simulink model "test"  (Simulink 7.5)
settings: Solver=ode45  StartTime=0.0  StopTime=10.0  RelTol=1e-3
libraries: neural x103
settings Model: Creator=SAM-PC  LastModifiedBy=SAM-PC

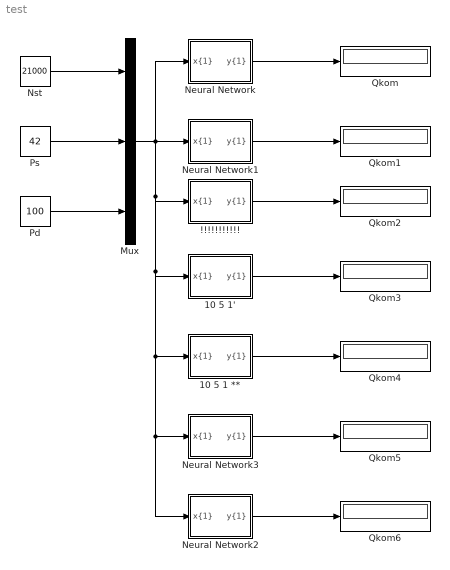
== system test ==
  !!!!!!!!!!! : Subsystem
  10 5 1 ** : Subsystem
  10 5 1' : Subsystem
  Mux : Mux  Inputs=3
  Neural Network : Subsystem
  Neural Network1 : Subsystem
  Neural Network2 : Subsystem
  Neural Network3 : Subsystem
  Nst : Constant  Value=21000  OutDataType=sfix(16)  OutScaling=2^0
  Pd : Constant  Value=100  OutDataType=sfix(16)  OutScaling=2^0
  Ps : Constant  Value=42  OutDataType=sfix(16)  OutScaling=2^0
  Qkom{,1..6} (7 alike) : Display
  wires:
  Mux/1 -> Neural Network/1("x{1}"), Neural Network1/1("x{1}"), !!!!!!!!!!!/1("x{1}"), 10 5 1'/1("x{1}"), 10 5 1 **/1("x{1}"), Neural Network3/1("x{1}"), Neural Network2/1("x{1}")
  Pd/1 -> Mux/3
  Ps/1 -> Mux/2
  Nst/1 -> Mux/1
  Neural Network/1("y{1}") -> Qkom/1
  Neural Network1/1("y{1}") -> Qkom1/1
  !!!!!!!!!!!/1("y{1}") -> Qkom2/1
  10 5 1'/1("y{1}") -> Qkom3/1
  10 5 1 **/1("y{1}") -> Qkom4/1
  Neural Network3/1("y{1}") -> Qkom5/1
  Neural Network2/1("y{1}") -> Qkom6/1

== system test/!!!!!!!!!!! ==
  "x{1}" : Inport  PortDimensions=3
  Layer 1 : Subsystem
  Layer 2 : Subsystem
  Process Input 1 : Subsystem
  Process Output 1 : Subsystem
  "y{1}" : Outport  InitialOutput=0
  wires:
  "x{1}"/1 -> Process Input 1/1(x)
  Process Output 1/1(y) -> "y{1}"/1
  Process Input 1/1(p) -> Layer 1/1("p{1}")
  Layer 1/1("a{1}") -> [feedback1]
  [feedback1] -> Layer 2/1("a{1} ")
  Layer 2/1("a{2}") -> Process Output 1/1(a)

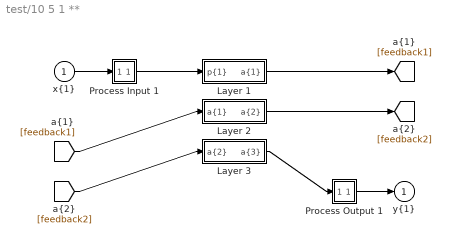
== system test/10 5 1 ** ==
  "x{1}" : Inport  PortDimensions=3
  Layer 1 : Subsystem
  Layer 2 : Subsystem
  Layer 3 : Subsystem
  Process Input 1 : Subsystem
  Process Output 1 : Subsystem
  "y{1}" : Outport  InitialOutput=0
  wires:
  Layer 3/1("a{3}") -> Process Output 1/1(a)
  [feedback2] -> Layer 3/1("a{2} ")
  Layer 2/1("a{2}") -> [feedback2]
  [feedback1] -> Layer 2/1("a{1} ")
  Layer 1/1("a{1}") -> [feedback1]
  Process Input 1/1(p) -> Layer 1/1("p{1}")
  Process Output 1/1(y) -> "y{1}"/1
  "x{1}"/1 -> Process Input 1/1(x)

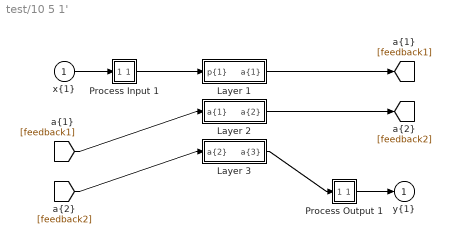
== system test/10 5 1' ==
  "x{1}" : Inport  PortDimensions=3
  Layer 1 : Subsystem
  Layer 2 : Subsystem
  Layer 3 : Subsystem
  Process Input 1 : Subsystem
  Process Output 1 : Subsystem
  "y{1}" : Outport  InitialOutput=0
  wires:
  Layer 3/1("a{3}") -> Process Output 1/1(a)
  [feedback2] -> Layer 3/1("a{2} ")
  Layer 2/1("a{2}") -> [feedback2]
  [feedback1] -> Layer 2/1("a{1} ")
  Layer 1/1("a{1}") -> [feedback1]
  Process Input 1/1(p) -> Layer 1/1("p{1}")
  Process Output 1/1(y) -> "y{1}"/1
  "x{1}"/1 -> Process Input 1/1(x)

== system test/Neural Network ==
  "x{1}" : Inport  PortDimensions=3
  Layer 1 : Subsystem
  Layer 2 : Subsystem
  Process Input 1 : Subsystem
  Process Output 1 : Subsystem
  "y{1}" : Outport  InitialOutput=0
  wires:
  "x{1}"/1 -> Process Input 1/1(x)
  Process Output 1/1(y) -> "y{1}"/1
  Process Input 1/1(p) -> Layer 1/1("p{1}")
  Layer 1/1("a{1}") -> [feedback1]
  [feedback1] -> Layer 2/1("a{1} ")
  Layer 2/1("a{2}") -> Process Output 1/1(a)

== system test/Neural Network1 ==
  "x{1}" : Inport  PortDimensions=3
  Layer 1 : Subsystem
  Layer 2 : Subsystem
  Process Input 1 : Subsystem
  Process Output 1 : Subsystem
  "y{1}" : Outport  InitialOutput=0
  wires:
  "x{1}"/1 -> Process Input 1/1(x)
  Process Output 1/1(y) -> "y{1}"/1
  Process Input 1/1(p) -> Layer 1/1("p{1}")
  Layer 1/1("a{1}") -> [feedback1]
  [feedback1] -> Layer 2/1("a{1} ")
  Layer 2/1("a{2}") -> Process Output 1/1(a)

== system test/Neural Network2 ==
  "x{1}" : Inport  PortDimensions=3
  Layer 1 : Subsystem
  Layer 2 : Subsystem
  Process Input 1 : Subsystem
  Process Output 1 : Subsystem
  "y{1}" : Outport  InitialOutput=0
  wires:
  Layer 2/1("a{2}") -> Process Output 1/1(a)
  [feedback1] -> Layer 2/1("a{1} ")
  Layer 1/1("a{1}") -> [feedback1]
  Process Input 1/1(p) -> Layer 1/1("p{1}")
  Process Output 1/1(y) -> "y{1}"/1
  "x{1}"/1 -> Process Input 1/1(x)

== system test/Neural Network3 ==
  "x{1}" : Inport  PortDimensions=3
  Layer 1 : Subsystem
  Layer 2 : Subsystem
  Process Input 1 : Subsystem
  Process Output 1 : Subsystem
  "y{1}" : Outport  InitialOutput=0
  wires:
  Layer 2/1("a{2}") -> Process Output 1/1(a)
  [feedback1] -> Layer 2/1("a{1} ")
  Layer 1/1("a{1}") -> [feedback1]
  Process Input 1/1(p) -> Layer 1/1("p{1}")
  Process Output 1/1(y) -> "y{1}"/1
  "x{1}"/1 -> Process Input 1/1(x)

== system test/!!!!!!!!!!!/Layer 1 ==
  "p{1}" : Inport  PortDimensions=3
  Delays 1 : Subsystem
      mask Display: disp('TDL')
  "IW{1,1}" : Subsystem
      mask Display: disp('weight')
  "b{1}" : Constant  Value=[-6.6059587578557615;-4.3526093218402542;-9.6125377715099489;15.34654034935151;-10.41504843932894;15.297045460594161;-11.215883022458025;-4.7902903485636283;-4.7770801252432253;-1.8726623455616338]
      mask Display: disp('bias')
  netsum : Sum  Inputs=2  OutDataType=sfix(16)  OutScaling=2^0  SaturateOnIntegerOverflow=on  InputSameDT=on  OutDataTypeStr=Inherit: Same as first input
  tansig : neural/Transfer Functions/tansig  SystemSampleTime=-1
  "a{1}" : Outport  InitialOutput=[0;0;0;0;0;0;0;0;0;0]
  wires:
  "p{1}"/1 -> Delays 1/1("p{1}")
  Delays 1/1("pd{1,1}") -> "IW{1,1}"/1("pd{1,1}")
  "IW{1,1}"/1("iz{1,1}") -> netsum/1
  "b{1}"/1 -> netsum/2
  netsum/1 -> tansig/1
  tansig/1 -> "a{1}"/1

== system test/!!!!!!!!!!!/Layer 2 ==
  "a{1} " : Inport  PortDimensions=10
  Delays 1 : Subsystem
      mask Display: disp('TDL')
  "LW{2,1}" : Subsystem
      mask Display: disp('weight')
  "b{2}" : Constant  Value=0.25321147312764225
      mask Display: disp('bias')
  netsum : Sum  Inputs=2  OutDataType=sfix(16)  OutScaling=2^0  SaturateOnIntegerOverflow=on  InputSameDT=on  OutDataTypeStr=Inherit: Same as first input
  purelin : neural/Transfer Functions/purelin  SystemSampleTime=-1
  "a{2}" : Outport  InitialOutput=0
  wires:
  "a{1} "/1 -> Delays 1/1("p{2}")
  Delays 1/1("pd{2,1}") -> "LW{2,1}"/1("ad{2,1}")
  "LW{2,1}"/1("lz{2,1}") -> netsum/1
  "b{2}"/1 -> netsum/2
  netsum/1 -> purelin/1
  purelin/1 -> "a{2}"/1

== system test/!!!!!!!!!!!/Process Input 1 ==
  x : Inport  PortDimensions=3
  p : Outport  PortDimensions=3
  wires:
  x/1 -> p/1

== system test/!!!!!!!!!!!/Process Output 1 ==
  a : Inport  PortDimensions=1
  y : Outport  PortDimensions=1
  wires:
  a/1 -> y/1

== system test/10 5 1 **/Layer 1 ==
  "p{1}" : Inport  PortDimensions=3
  Delays 1 : Subsystem
      mask Display: disp('TDL')
  "IW{1,1}" : Subsystem
      mask Display: disp('weight')
  "b{1}" : Constant  Value=[15.02277102392976;-1.3070946494642188;25.056968170821065;1.5453975487445806;-0.48029688944254451;5.9693538654521783;7.7677013128534886;-4.9232036490574114;-12.41463739376492;0.1231144148821651]
      mask Display: disp('bias')
  netsum : Sum  Inputs=2  OutDataType=sfix(16)  OutScaling=2^0  SaturateOnIntegerOverflow=on  InputSameDT=on  OutDataTypeStr=Inherit: Same as first input
  tansig : neural/Transfer Functions/tansig  SystemSampleTime=-1
  "a{1}" : Outport  InitialOutput=[0;0;0;0;0;0;0;0;0;0]
  wires:
  tansig/1 -> "a{1}"/1
  netsum/1 -> tansig/1
  "b{1}"/1 -> netsum/2
  "IW{1,1}"/1("iz{1,1}") -> netsum/1
  Delays 1/1("pd{1,1}") -> "IW{1,1}"/1("pd{1,1}")
  "p{1}"/1 -> Delays 1/1("p{1}")

== system test/10 5 1 **/Layer 2 ==
  "a{1} " : Inport  PortDimensions=10
  Delays 1 : Subsystem
      mask Display: disp('TDL')
  "LW{2,1}" : Subsystem
      mask Display: disp('weight')
  "b{2}" : Constant  Value=[2.8247030289932828;-7.9344890622783693;-8.5564708148276107;2.9733715127865676;6.28273195654105]
      mask Display: disp('bias')
  netsum : Sum  Inputs=2  OutDataType=sfix(16)  OutScaling=2^0  SaturateOnIntegerOverflow=on  InputSameDT=on  OutDataTypeStr=Inherit: Same as first input
  tansig : neural/Transfer Functions/tansig  SystemSampleTime=-1
  "a{2}" : Outport  InitialOutput=[0;0;0;0;0]
  wires:
  tansig/1 -> "a{2}"/1
  netsum/1 -> tansig/1
  "b{2}"/1 -> netsum/2
  "LW{2,1}"/1("lz{2,1}") -> netsum/1
  Delays 1/1("pd{2,1}") -> "LW{2,1}"/1("ad{2,1}")
  "a{1} "/1 -> Delays 1/1("p{2}")

== system test/10 5 1 **/Layer 3 ==
  "a{2} " : Inport  PortDimensions=5
  Delays 1 : Subsystem
      mask Display: disp('TDL')
  "LW{3,2}" : Subsystem
      mask Display: disp('weight')
  "b{3}" : Constant  Value=0.30034208922808647
      mask Display: disp('bias')
  netsum : Sum  Inputs=2  OutDataType=sfix(16)  OutScaling=2^0  SaturateOnIntegerOverflow=on  InputSameDT=on  OutDataTypeStr=Inherit: Same as first input
  purelin : neural/Transfer Functions/purelin  SystemSampleTime=-1
  "a{3}" : Outport  InitialOutput=0
  wires:
  purelin/1 -> "a{3}"/1
  netsum/1 -> purelin/1
  "b{3}"/1 -> netsum/2
  "LW{3,2}"/1("lz{3,2}") -> netsum/1
  Delays 1/1("pd{3,2}") -> "LW{3,2}"/1("ad{3,2}")
  "a{2} "/1 -> Delays 1/1("p{3}")

== system test/10 5 1 **/Process Input 1 ==
  x : Inport  PortDimensions=3
  p : Outport  PortDimensions=3
  wires:
  x/1 -> p/1

== system test/10 5 1 **/Process Output 1 ==
  a : Inport  PortDimensions=1
  y : Outport  PortDimensions=1
  wires:
  a/1 -> y/1

== system test/10 5 1'/Layer 1 ==
  "p{1}" : Inport  PortDimensions=3
  Delays 1 : Subsystem
      mask Display: disp('TDL')
  "IW{1,1}" : Subsystem
      mask Display: disp('weight')
  "b{1}" : Constant  Value=[18.413579066262386;13.657316243075135;18.043767679185159;11.250334678262735;3.5241900842698204;13.404243407569995;2.2257807010437509;9.6566319022558904;-3.0274634325673926;-4.0023507151100919]
      mask Display: disp('bias')
  netsum : Sum  Inputs=2  OutDataType=sfix(16)  OutScaling=2^0  SaturateOnIntegerOverflow=on  InputSameDT=on  OutDataTypeStr=Inherit: Same as first input
  tansig : neural/Transfer Functions/tansig  SystemSampleTime=-1
  "a{1}" : Outport  InitialOutput=[0;0;0;0;0;0;0;0;0;0]
  wires:
  tansig/1 -> "a{1}"/1
  netsum/1 -> tansig/1
  "b{1}"/1 -> netsum/2
  "IW{1,1}"/1("iz{1,1}") -> netsum/1
  Delays 1/1("pd{1,1}") -> "IW{1,1}"/1("pd{1,1}")
  "p{1}"/1 -> Delays 1/1("p{1}")

== system test/10 5 1'/Layer 2 ==
  "a{1} " : Inport  PortDimensions=10
  Delays 1 : Subsystem
      mask Display: disp('TDL')
  "LW{2,1}" : Subsystem
      mask Display: disp('weight')
  "b{2}" : Constant  Value=[2.1532494058916414;-0.67401500656272084;0.59110621272557129;-0.67490370527186982;1.3792550590079387]
      mask Display: disp('bias')
  netsum : Sum  Inputs=2  OutDataType=sfix(16)  OutScaling=2^0  SaturateOnIntegerOverflow=on  InputSameDT=on  OutDataTypeStr=Inherit: Same as first input
  tansig : neural/Transfer Functions/tansig  SystemSampleTime=-1
  "a{2}" : Outport  InitialOutput=[0;0;0;0;0]
  wires:
  tansig/1 -> "a{2}"/1
  netsum/1 -> tansig/1
  "b{2}"/1 -> netsum/2
  "LW{2,1}"/1("lz{2,1}") -> netsum/1
  Delays 1/1("pd{2,1}") -> "LW{2,1}"/1("ad{2,1}")
  "a{1} "/1 -> Delays 1/1("p{2}")

== system test/10 5 1'/Layer 3 ==
  "a{2} " : Inport  PortDimensions=5
  Delays 1 : Subsystem
      mask Display: disp('TDL')
  "LW{3,2}" : Subsystem
      mask Display: disp('weight')
  "b{3}" : Constant  Value=1.1366411649250561
      mask Display: disp('bias')
  netsum : Sum  Inputs=2  OutDataType=sfix(16)  OutScaling=2^0  SaturateOnIntegerOverflow=on  InputSameDT=on  OutDataTypeStr=Inherit: Same as first input
  purelin : neural/Transfer Functions/purelin  SystemSampleTime=-1
  "a{3}" : Outport  InitialOutput=0
  wires:
  purelin/1 -> "a{3}"/1
  netsum/1 -> purelin/1
  "b{3}"/1 -> netsum/2
  "LW{3,2}"/1("lz{3,2}") -> netsum/1
  Delays 1/1("pd{3,2}") -> "LW{3,2}"/1("ad{3,2}")
  "a{2} "/1 -> Delays 1/1("p{3}")

== system test/10 5 1'/Process Input 1 ==
  x : Inport  PortDimensions=3
  p : Outport  PortDimensions=3
  wires:
  x/1 -> p/1

== system test/10 5 1'/Process Output 1 ==
  a : Inport  PortDimensions=1
  y : Outport  PortDimensions=1
  wires:
  a/1 -> y/1

== system test/Neural Network/Layer 1 ==
  "p{1}" : Inport  PortDimensions=3
  Delays 1 : Subsystem
      mask Display: disp('TDL')
  "IW{1,1}" : Subsystem
      mask Display: disp('weight')
  "b{1}" : Constant  Value=[2.4324708557605383;-7.6739421539174089;3.0539465468465736;18.55085646224725;-23.635141756656115;-2.6793611692857526;17.680290988578996;-14.569548932519789;-13.842527653317914;-3.4475580624121687]
      mask Display: disp('bias')
  netsum : Sum  Inputs=2  OutDataType=sfix(16)  OutScaling=2^0  SaturateOnIntegerOverflow=on  InputSameDT=on  OutDataTypeStr=Inherit: Same as first input
  tansig : neural/Transfer Functions/tansig  SystemSampleTime=-1
  "a{1}" : Outport  InitialOutput=[0;0;0;0;0;0;0;0;0;0]
  wires:
  "p{1}"/1 -> Delays 1/1("p{1}")
  Delays 1/1("pd{1,1}") -> "IW{1,1}"/1("pd{1,1}")
  "IW{1,1}"/1("iz{1,1}") -> netsum/1
  "b{1}"/1 -> netsum/2
  netsum/1 -> tansig/1
  tansig/1 -> "a{1}"/1

== system test/Neural Network/Layer 2 ==
  "a{1} " : Inport  PortDimensions=10
  Delays 1 : Subsystem
      mask Display: disp('TDL')
  "LW{2,1}" : Subsystem
      mask Display: disp('weight')
  "b{2}" : Constant  Value=0.15810922780423164
      mask Display: disp('bias')
  netsum : Sum  Inputs=2  OutDataType=sfix(16)  OutScaling=2^0  SaturateOnIntegerOverflow=on  InputSameDT=on  OutDataTypeStr=Inherit: Same as first input
  purelin : neural/Transfer Functions/purelin  SystemSampleTime=-1
  "a{2}" : Outport  InitialOutput=0
  wires:
  "a{1} "/1 -> Delays 1/1("p{2}")
  Delays 1/1("pd{2,1}") -> "LW{2,1}"/1("ad{2,1}")
  "LW{2,1}"/1("lz{2,1}") -> netsum/1
  "b{2}"/1 -> netsum/2
  netsum/1 -> purelin/1
  purelin/1 -> "a{2}"/1

== system test/Neural Network/Process Input 1 ==
  x : Inport  PortDimensions=3
  p : Outport  PortDimensions=3
  wires:
  x/1 -> p/1

== system test/Neural Network/Process Output 1 ==
  a : Inport  PortDimensions=1
  y : Outport  PortDimensions=1
  wires:
  a/1 -> y/1

== system test/Neural Network1/Layer 1 ==
  "p{1}" : Inport  PortDimensions=3
  Delays 1 : Subsystem
      mask Display: disp('TDL')
  "IW{1,1}" : Subsystem
      mask Display: disp('weight')
  "b{1}" : Constant  Value=[-6.0166931774834991;-46.688706694529984;5.2999690825438703;18.493444026928799;-18.348040178794896;2.6103626315712543;-18.12090596934063;-7.1161048627161625;6.9740359095450248;-8.6996750974869972]
      mask Display: disp('bias')
  netsum : Sum  Inputs=2  OutDataType=sfix(16)  OutScaling=2^0  SaturateOnIntegerOverflow=on  InputSameDT=on  OutDataTypeStr=Inherit: Same as first input
  tansig : neural/Transfer Functions/tansig  SystemSampleTime=-1
  "a{1}" : Outport  InitialOutput=[0;0;0;0;0;0;0;0;0;0]
  wires:
  "p{1}"/1 -> Delays 1/1("p{1}")
  Delays 1/1("pd{1,1}") -> "IW{1,1}"/1("pd{1,1}")
  "IW{1,1}"/1("iz{1,1}") -> netsum/1
  "b{1}"/1 -> netsum/2
  netsum/1 -> tansig/1
  tansig/1 -> "a{1}"/1

== system test/Neural Network1/Layer 2 ==
  "a{1} " : Inport  PortDimensions=10
  Delays 1 : Subsystem
      mask Display: disp('TDL')
  "LW{2,1}" : Subsystem
      mask Display: disp('weight')
  "b{2}" : Constant  Value=-0.029512269905579976
      mask Display: disp('bias')
  netsum : Sum  Inputs=2  OutDataType=sfix(16)  OutScaling=2^0  SaturateOnIntegerOverflow=on  InputSameDT=on  OutDataTypeStr=Inherit: Same as first input
  purelin : neural/Transfer Functions/purelin  SystemSampleTime=-1
  "a{2}" : Outport  InitialOutput=0
  wires:
  "a{1} "/1 -> Delays 1/1("p{2}")
  Delays 1/1("pd{2,1}") -> "LW{2,1}"/1("ad{2,1}")
  "LW{2,1}"/1("lz{2,1}") -> netsum/1
  "b{2}"/1 -> netsum/2
  netsum/1 -> purelin/1
  purelin/1 -> "a{2}"/1

== system test/Neural Network1/Process Input 1 ==
  x : Inport  PortDimensions=3
  p : Outport  PortDimensions=3
  wires:
  x/1 -> p/1

== system test/Neural Network1/Process Output 1 ==
  a : Inport  PortDimensions=1
  y : Outport  PortDimensions=1
  wires:
  a/1 -> y/1

== system test/Neural Network2/Layer 1 ==
  "p{1}" : Inport  PortDimensions=3
  Delays 1 : Subsystem
      mask Display: disp('TDL')
  "IW{1,1}" : Subsystem
      mask Display: disp('weight')
  "b{1}" : Constant  Value=[15.912206318753258;7.7505120175037128;3.9018047854873212;-15.426996139049765;2.823989991488741;-11.93381184712964;-15.394961107894558;1.9154713229925484;-8.9241881256300211;-7.3222794371491178]
      mask Display: disp('bias')
  netsum : Sum  Inputs=2  OutDataType=sfix(16)  OutScaling=2^0  SaturateOnIntegerOverflow=on  InputSameDT=on  OutDataTypeStr=Inherit: Same as first input
  tansig : neural/Transfer Functions/tansig  SystemSampleTime=-1
  "a{1}" : Outport  InitialOutput=[0;0;0;0;0;0;0;0;0;0]
  wires:
  tansig/1 -> "a{1}"/1
  netsum/1 -> tansig/1
  "b{1}"/1 -> netsum/2
  "IW{1,1}"/1("iz{1,1}") -> netsum/1
  Delays 1/1("pd{1,1}") -> "IW{1,1}"/1("pd{1,1}")
  "p{1}"/1 -> Delays 1/1("p{1}")

== system test/Neural Network2/Layer 2 ==
  "a{1} " : Inport  PortDimensions=10
  Delays 1 : Subsystem
      mask Display: disp('TDL')
  "LW{2,1}" : Subsystem
      mask Display: disp('weight')
  "b{2}" : Constant  Value=0.97737461588991392
      mask Display: disp('bias')
  netsum : Sum  Inputs=2  OutDataType=sfix(16)  OutScaling=2^0  SaturateOnIntegerOverflow=on  InputSameDT=on  OutDataTypeStr=Inherit: Same as first input
  purelin : neural/Transfer Functions/purelin  SystemSampleTime=-1
  "a{2}" : Outport  InitialOutput=0
  wires:
  purelin/1 -> "a{2}"/1
  netsum/1 -> purelin/1
  "b{2}"/1 -> netsum/2
  "LW{2,1}"/1("lz{2,1}") -> netsum/1
  Delays 1/1("pd{2,1}") -> "LW{2,1}"/1("ad{2,1}")
  "a{1} "/1 -> Delays 1/1("p{2}")

== system test/Neural Network2/Process Input 1 ==
  x : Inport  PortDimensions=3
  p : Outport  PortDimensions=3
  wires:
  x/1 -> p/1

== system test/Neural Network2/Process Output 1 ==
  a : Inport  PortDimensions=1
  y : Outport  PortDimensions=1
  wires:
  a/1 -> y/1

== system test/Neural Network3/Layer 1 ==
  "p{1}" : Inport  PortDimensions=3
  Delays 1 : Subsystem
      mask Display: disp('TDL')
  "IW{1,1}" : Subsystem
      mask Display: disp('weight')
  "b{1}" : Constant  Value=[-22.415234115254385;-11.362832743815702;13.196213345352477;-23.274128799542019;-1.9079448236650758;5.6206820240612299;-14.499132702291242;-18.316509525440882;-16.167922059318332;-12.536388092109599]
      mask Display: disp('bias')
  netsum : Sum  Inputs=2  OutDataType=sfix(16)  OutScaling=2^0  SaturateOnIntegerOverflow=on  InputSameDT=on  OutDataTypeStr=Inherit: Same as first input
  tansig : neural/Transfer Functions/tansig  SystemSampleTime=-1
  "a{1}" : Outport  InitialOutput=[0;0;0;0;0;0;0;0;0;0]
  wires:
  tansig/1 -> "a{1}"/1
  netsum/1 -> tansig/1
  "b{1}"/1 -> netsum/2
  "IW{1,1}"/1("iz{1,1}") -> netsum/1
  Delays 1/1("pd{1,1}") -> "IW{1,1}"/1("pd{1,1}")
  "p{1}"/1 -> Delays 1/1("p{1}")

== system test/Neural Network3/Layer 2 ==
  "a{1} " : Inport  PortDimensions=10
  Delays 1 : Subsystem
      mask Display: disp('TDL')
  "LW{2,1}" : Subsystem
      mask Display: disp('weight')
  "b{2}" : Constant  Value=1.0819192782537284
      mask Display: disp('bias')
  netsum : Sum  Inputs=2  OutDataType=sfix(16)  OutScaling=2^0  SaturateOnIntegerOverflow=on  InputSameDT=on  OutDataTypeStr=Inherit: Same as first input
  purelin : neural/Transfer Functions/purelin  SystemSampleTime=-1
  "a{2}" : Outport  InitialOutput=0
  wires:
  purelin/1 -> "a{2}"/1
  netsum/1 -> purelin/1
  "b{2}"/1 -> netsum/2
  "LW{2,1}"/1("lz{2,1}") -> netsum/1
  Delays 1/1("pd{2,1}") -> "LW{2,1}"/1("ad{2,1}")
  "a{1} "/1 -> Delays 1/1("p{2}")

== system test/Neural Network3/Process Input 1 ==
  x : Inport  PortDimensions=3
  p : Outport  PortDimensions=3
  wires:
  x/1 -> p/1

== system test/Neural Network3/Process Output 1 ==
  a : Inport  PortDimensions=1
  y : Outport  PortDimensions=1
  wires:
  a/1 -> y/1

== system test/!!!!!!!!!!!/Layer 1/Delays 1 ==
  "p{1}" : Inport  PortDimensions=3
  mux : Mux  Inputs=1
  "pd{1,1}" : Outport
  wires:
  "p{1}"/1 -> mux/1
  mux/1 -> "pd{1,1}"/1

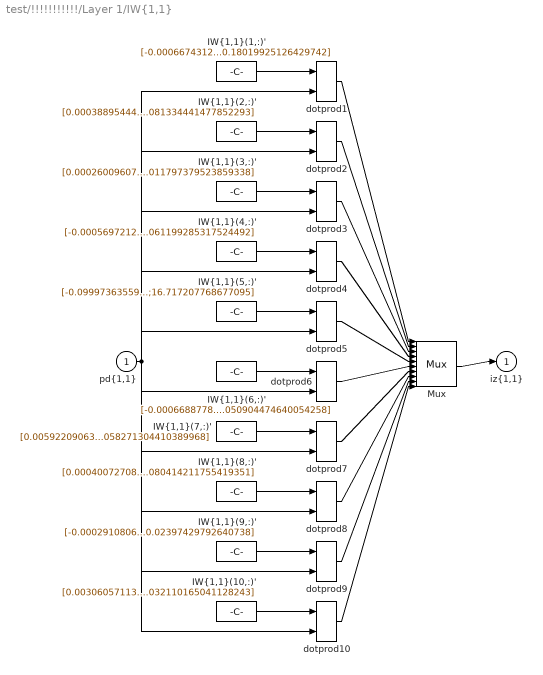
== system test/!!!!!!!!!!!/Layer 1/IW{1,1} ==
  "pd{1,1}" : Inport  PortDimensions=3
  "IW{1,1}(1,:)'" : Constant  Value=[-0.00066743122035897099;-0.11206446014488511;0.18019925126429742]
      mask Display: disp('weights')
  "IW{1,1}(10,:)'" : Constant  Value=[0.0030605711313751579;-0.096052630538237732;-0.032110165041128243]
      mask Display: disp('weights')
  "IW{1,1}(2,:)'" : Constant  Value=[0.0003889544485913661;0.15069729232506487;-0.081334441477852293]
      mask Display: disp('weights')
  "IW{1,1}(3,:)'" : Constant  Value=[0.00026009607440958632;0.063526490616979098;0.011797379523859338]
      mask Display: disp('weights')
  "IW{1,1}(4,:)'" : Constant  Value=[-0.00056972120462246755;-0.19132461828198041;0.061199285317524492]
      mask Display: disp('weights')
  "IW{1,1}(5,:)'" : Constant  Value=[-0.099973635598832711;2.8634131297756991;16.717207768677095]
      mask Display: disp('weights')
  "IW{1,1}(6,:)'" : Constant  Value=[-0.00066887787432494861;-0.18010598749241391;0.050904474640054258]
      mask Display: disp('weights')
  "IW{1,1}(7,:)'" : Constant  Value=[0.0059220906350217883;0.11468973909442041;-0.0058271304410389968]
      mask Display: disp('weights')
  "IW{1,1}(8,:)'" : Constant  Value=[0.00040072708699105176;0.15224871553489033;-0.080414211755419351]
      mask Display: disp('weights')
  "IW{1,1}(9,:)'" : Constant  Value=[-0.00029108067581634574;0.221865316933716;0.02397429792640738]
      mask Display: disp('weights')
  Mux : Mux  Inputs=10
  dotprod{1..10} (10 alike) : neural/Weight Functions/dotprod  SystemSampleTime=-1
  "iz{1,1}" : Outport
  wires:
  "IW{1,1}(1,:)'"/1 -> dotprod1/1
  "pd{1,1}"/1 -> dotprod1/2, dotprod2/2, dotprod3/2, dotprod4/2, dotprod5/2, dotprod6/2, dotprod7/2, dotprod8/2, dotprod9/2, dotprod10/2
  dotprod1/1 -> Mux/1
  "IW{1,1}(2,:)'"/1 -> dotprod2/1
  dotprod2/1 -> Mux/2
  "IW{1,1}(3,:)'"/1 -> dotprod3/1
  dotprod3/1 -> Mux/3
  "IW{1,1}(4,:)'"/1 -> dotprod4/1
  dotprod4/1 -> Mux/4
  "IW{1,1}(5,:)'"/1 -> dotprod5/1
  dotprod5/1 -> Mux/5
  "IW{1,1}(6,:)'"/1 -> dotprod6/1
  dotprod6/1 -> Mux/6
  "IW{1,1}(7,:)'"/1 -> dotprod7/1
  dotprod7/1 -> Mux/7
  "IW{1,1}(8,:)'"/1 -> dotprod8/1
  dotprod8/1 -> Mux/8
  "IW{1,1}(9,:)'"/1 -> dotprod9/1
  dotprod9/1 -> Mux/9
  "IW{1,1}(10,:)'"/1 -> dotprod10/1
  dotprod10/1 -> Mux/10
  Mux/1 -> "iz{1,1}"/1

== system test/!!!!!!!!!!!/Layer 2/Delays 1 ==
  "p{2}" : Inport  PortDimensions=10
  mux : Mux  Inputs=1
  "pd{2,1}" : Outport
  wires:
  "p{2}"/1 -> mux/1
  mux/1 -> "pd{2,1}"/1

== system test/!!!!!!!!!!!/Layer 2/LW{2,1} ==
  "ad{2,1}" : Inport  PortDimensions=10
  "IW{2,1}(1,:)'" : Constant  Value=[0.2014952594481072;-17.665856907001295;0.32895145996666803;-0.16313906729449315;-0.010968372198123189;-0.16608301452374061;0.4906858391457794;18.608278949900093;0.057164287403765564;-0.050891845936561014]
      mask Display: disp('weights')
  Mux : Mux  Inputs=1
  dotprod1 : neural/Weight Functions/dotprod  SystemSampleTime=-1
  "lz{2,1}" : Outport
  wires:
  "IW{2,1}(1,:)'"/1 -> dotprod1/1
  "ad{2,1}"/1 -> dotprod1/2
  dotprod1/1 -> Mux/1
  Mux/1 -> "lz{2,1}"/1

== system test/10 5 1 **/Layer 1/Delays 1 ==
  "p{1}" : Inport  PortDimensions=3
  mux : Mux  Inputs=1
  "pd{1,1}" : Outport
  wires:
  mux/1 -> "pd{1,1}"/1
  "p{1}"/1 -> mux/1

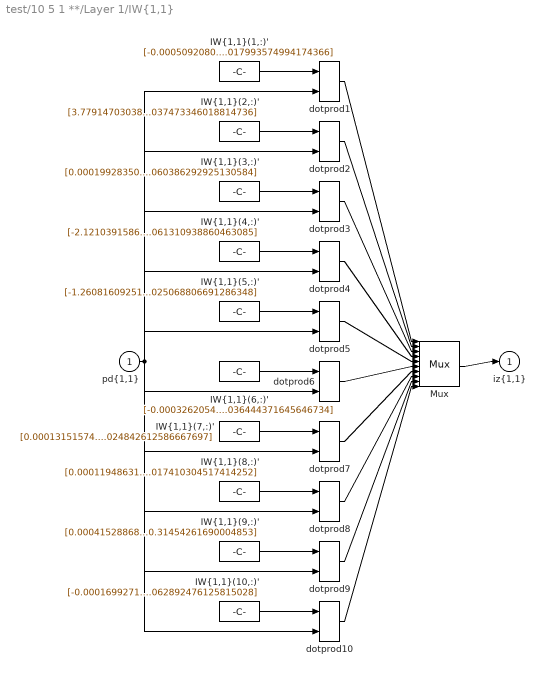
== system test/10 5 1 **/Layer 1/IW{1,1} ==
  "pd{1,1}" : Inport  PortDimensions=3
  "IW{1,1}(1,:)'" : Constant  Value=[-0.00050920807284234569;-0.0085213186599955425;-0.017993574994174366]
      mask Display: disp('weights')
  "IW{1,1}(10,:)'" : Constant  Value=[-0.00016992715816369633;-0.10972561846862412;0.062892476125815028]
      mask Display: disp('weights')
  "IW{1,1}(2,:)'" : Constant  Value=[3.7791470303831908e-005;0.0018724309545801534;0.0037473346018814736]
      mask Display: disp('weights')
  "IW{1,1}(3,:)'" : Constant  Value=[0.00019928350232927751;-0.82151421566884497;0.060386292925130584]
      mask Display: disp('weights')
  "IW{1,1}(4,:)'" : Constant  Value=[-2.121039158636167e-005;-0.078980950618775914;0.061310938860463085]
      mask Display: disp('weights')
  "IW{1,1}(5,:)'" : Constant  Value=[-1.2608160925138492e-005;-0.023998321994299732;0.0025068806691286348]
      mask Display: disp('weights')
  "IW{1,1}(6,:)'" : Constant  Value=[-0.00032620549407861248;-0.08319477794048076;0.036444371645646734]
      mask Display: disp('weights')
  "IW{1,1}(7,:)'" : Constant  Value=[0.00013151574843368863;-0.30850562387531805;0.024842612586667697]
      mask Display: disp('weights')
  "IW{1,1}(8,:)'" : Constant  Value=[0.00011948631518652662;0.0094847284701925459;0.017410304517414252]
      mask Display: disp('weights')
  "IW{1,1}(9,:)'" : Constant  Value=[0.00041528868369263781;1.1057605566848399;-0.31454261690004853]
      mask Display: disp('weights')
  Mux : Mux  Inputs=10
  dotprod{1..10} (10 alike) : neural/Weight Functions/dotprod  SystemSampleTime=-1
  "iz{1,1}" : Outport
  wires:
  Mux/1 -> "iz{1,1}"/1
  dotprod10/1 -> Mux/10
  "IW{1,1}(10,:)'"/1 -> dotprod10/1
  dotprod9/1 -> Mux/9
  "IW{1,1}(9,:)'"/1 -> dotprod9/1
  dotprod8/1 -> Mux/8
  "IW{1,1}(8,:)'"/1 -> dotprod8/1
  dotprod7/1 -> Mux/7
  "IW{1,1}(7,:)'"/1 -> dotprod7/1
  dotprod6/1 -> Mux/6
  "IW{1,1}(6,:)'"/1 -> dotprod6/1
  dotprod5/1 -> Mux/5
  "IW{1,1}(5,:)'"/1 -> dotprod5/1
  dotprod4/1 -> Mux/4
  "IW{1,1}(4,:)'"/1 -> dotprod4/1
  dotprod3/1 -> Mux/3
  "IW{1,1}(3,:)'"/1 -> dotprod3/1
  dotprod2/1 -> Mux/2
  "IW{1,1}(2,:)'"/1 -> dotprod2/1
  dotprod1/1 -> Mux/1
  "pd{1,1}"/1 -> dotprod10/2, dotprod9/2, dotprod8/2, dotprod7/2, dotprod6/2, dotprod5/2, dotprod4/2, dotprod3/2, dotprod2/2, dotprod1/2
  "IW{1,1}(1,:)'"/1 -> dotprod1/1

== system test/10 5 1 **/Layer 2/Delays 1 ==
  "p{2}" : Inport  PortDimensions=10
  mux : Mux  Inputs=1
  "pd{2,1}" : Outport
  wires:
  mux/1 -> "pd{2,1}"/1
  "p{2}"/1 -> mux/1

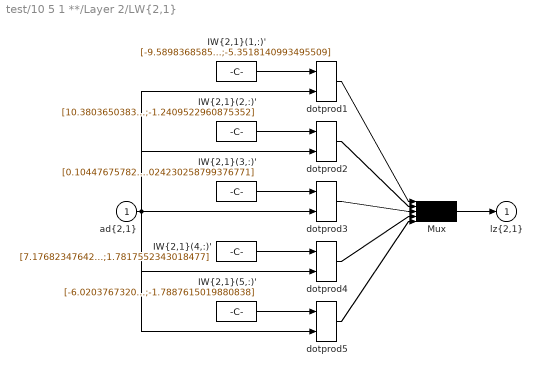
== system test/10 5 1 **/Layer 2/LW{2,1} ==
  "ad{2,1}" : Inport  PortDimensions=10
  "IW{2,1}(1,:)'" : Constant  Value=[-9.5898368585570974;0.49899884640485281;-0.0050039404653001414;-0.065234216891695285;0.25337329235477291;0.14130594589974615;0.033977305942516932;1.7590127386237366;4.4883974553013468;-5.3518140993495509]
      mask Display: disp('weights')
  "IW{2,1}(2,:)'" : Constant  Value=[10.380365038321104;-2.2736544041010998;-1.2759562227948249;-1.4508284627141894;-5.0489569371074028;-11.415353348591724;2.4885526520364163;-1.2311835440957277;-3.4493422275034651;-1.2409522960875352]
      mask Display: disp('weights')
  "IW{2,1}(3,:)'" : Constant  Value=[0.10447675782041345;3.0725539305373464;-0.021828632228172801;-0.19408376411603948;-4.5368938638238614;-0.13615111962573198;0.047613767717078079;-0.58727849664091503;3.6135738347819619;-0.024230258799376771]
      mask Display: disp('weights')
  "IW{2,1}(4,:)'" : Constant  Value=[7.1768234764234284;19.0921657841462;1.4005172899896623;4.4884737090141771;-5.0603875861965477;-5.4077482335169353;4.4663399667615211;5.4016505505261252;5.149488234094572;1.7817552343018477]
      mask Display: disp('weights')
  "IW{2,1}(5,:)'" : Constant  Value=[-6.0203767320220516;-13.339528090560707;0.28370059186492791;0.18491240480515703;3.5091859651398067;-3.540932485795663;-0.56598200446423741;3.802736193308053;2.1740599947842685;-1.7887615019880838]
      mask Display: disp('weights')
  Mux : Mux  Inputs=5
  dotprod{1..5} (5 alike) : neural/Weight Functions/dotprod  SystemSampleTime=-1
  "lz{2,1}" : Outport
  wires:
  Mux/1 -> "lz{2,1}"/1
  dotprod5/1 -> Mux/5
  "IW{2,1}(5,:)'"/1 -> dotprod5/1
  dotprod4/1 -> Mux/4
  "IW{2,1}(4,:)'"/1 -> dotprod4/1
  dotprod3/1 -> Mux/3
  "IW{2,1}(3,:)'"/1 -> dotprod3/1
  dotprod2/1 -> Mux/2
  "IW{2,1}(2,:)'"/1 -> dotprod2/1
  dotprod1/1 -> Mux/1
  "ad{2,1}"/1 -> dotprod5/2, dotprod4/2, dotprod3/2, dotprod2/2, dotprod1/2
  "IW{2,1}(1,:)'"/1 -> dotprod1/1

== system test/10 5 1 **/Layer 3/Delays 1 ==
  "p{3}" : Inport  PortDimensions=5
  mux : Mux  Inputs=1
  "pd{3,2}" : Outport
  wires:
  mux/1 -> "pd{3,2}"/1
  "p{3}"/1 -> mux/1

== system test/10 5 1 **/Layer 3/LW{3,2} ==
  "ad{3,2}" : Inport  PortDimensions=5
  "IW{3,2}(1,:)'" : Constant  Value=[-2.5588530966053775;0.016276628658331672;5.1009656353719679;-0.51744224066969813;7.529504795175348]
      mask Display: disp('weights')
  Mux : Mux  Inputs=1
  dotprod1 : neural/Weight Functions/dotprod  SystemSampleTime=-1
  "lz{3,2}" : Outport
  wires:
  Mux/1 -> "lz{3,2}"/1
  dotprod1/1 -> Mux/1
  "ad{3,2}"/1 -> dotprod1/2
  "IW{3,2}(1,:)'"/1 -> dotprod1/1

== system test/10 5 1'/Layer 1/Delays 1 ==
  "p{1}" : Inport  PortDimensions=3
  mux : Mux  Inputs=1
  "pd{1,1}" : Outport
  wires:
  mux/1 -> "pd{1,1}"/1
  "p{1}"/1 -> mux/1

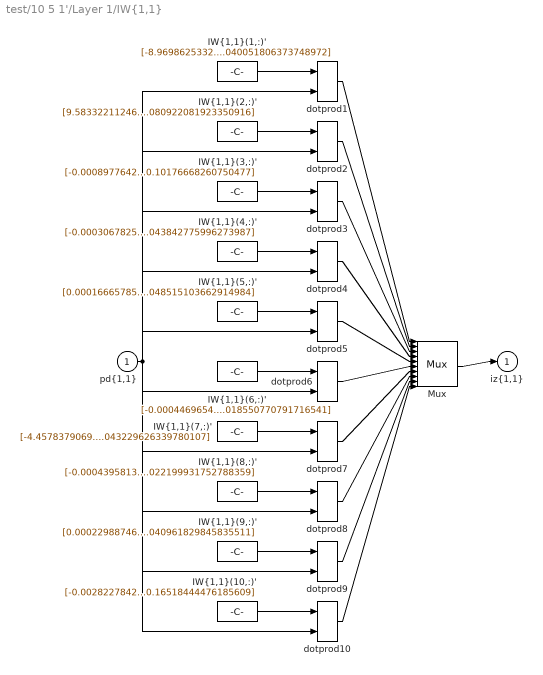
== system test/10 5 1'/Layer 1/IW{1,1} ==
  "pd{1,1}" : Inport  PortDimensions=3
  "IW{1,1}(1,:)'" : Constant  Value=[-8.9698625332169449e-005;-0.2777959474969936;-0.040051806373748972]
      mask Display: disp('weights')
  "IW{1,1}(10,:)'" : Constant  Value=[-0.0028227842061574809;0.87051129609929689;-0.16518444476185609]
      mask Display: disp('weights')
  "IW{1,1}(2,:)'" : Constant  Value=[9.5833221124630503e-005;-0.27272693821077809;-0.080922081923350916]
      mask Display: disp('weights')
  "IW{1,1}(3,:)'" : Constant  Value=[-0.00089776424560656363;-0.26478304808332526;0.10176668260750477]
      mask Display: disp('weights')
  "IW{1,1}(4,:)'" : Constant  Value=[-0.00030678252369395058;-0.22816738972766309;0.043842775996273987]
      mask Display: disp('weights')
  "IW{1,1}(5,:)'" : Constant  Value=[0.00016665785128819257;-0.2088209823102315;0.048515103662914984]
      mask Display: disp('weights')
  "IW{1,1}(6,:)'" : Constant  Value=[-0.00044696547274784387;-0.12095789757637422;0.018550770791716541]
      mask Display: disp('weights')
  "IW{1,1}(7,:)'" : Constant  Value=[-4.4578379069228317e-005;0.097076251254256729;-0.043229626339780107]
      mask Display: disp('weights')
  "IW{1,1}(8,:)'" : Constant  Value=[-0.0004395813619963683;-0.012840297613209636;-0.022199931752788359]
      mask Display: disp('weights')
  "IW{1,1}(9,:)'" : Constant  Value=[0.00022988746228307894;0.050529283752709077;-0.040961829845835511]
      mask Display: disp('weights')
  Mux : Mux  Inputs=10
  dotprod{1..10} (10 alike) : neural/Weight Functions/dotprod  SystemSampleTime=-1
  "iz{1,1}" : Outport
  wires:
  Mux/1 -> "iz{1,1}"/1
  dotprod10/1 -> Mux/10
  "IW{1,1}(10,:)'"/1 -> dotprod10/1
  dotprod9/1 -> Mux/9
  "IW{1,1}(9,:)'"/1 -> dotprod9/1
  dotprod8/1 -> Mux/8
  "IW{1,1}(8,:)'"/1 -> dotprod8/1
  dotprod7/1 -> Mux/7
  "IW{1,1}(7,:)'"/1 -> dotprod7/1
  dotprod6/1 -> Mux/6
  "IW{1,1}(6,:)'"/1 -> dotprod6/1
  dotprod5/1 -> Mux/5
  "IW{1,1}(5,:)'"/1 -> dotprod5/1
  dotprod4/1 -> Mux/4
  "IW{1,1}(4,:)'"/1 -> dotprod4/1
  dotprod3/1 -> Mux/3
  "IW{1,1}(3,:)'"/1 -> dotprod3/1
  dotprod2/1 -> Mux/2
  "IW{1,1}(2,:)'"/1 -> dotprod2/1
  dotprod1/1 -> Mux/1
  "pd{1,1}"/1 -> dotprod10/2, dotprod9/2, dotprod8/2, dotprod7/2, dotprod6/2, dotprod5/2, dotprod4/2, dotprod3/2, dotprod2/2, dotprod1/2
  "IW{1,1}(1,:)'"/1 -> dotprod1/1

== system test/10 5 1'/Layer 2/Delays 1 ==
  "p{2}" : Inport  PortDimensions=10
  mux : Mux  Inputs=1
  "pd{2,1}" : Outport
  wires:
  mux/1 -> "pd{2,1}"/1
  "p{2}"/1 -> mux/1

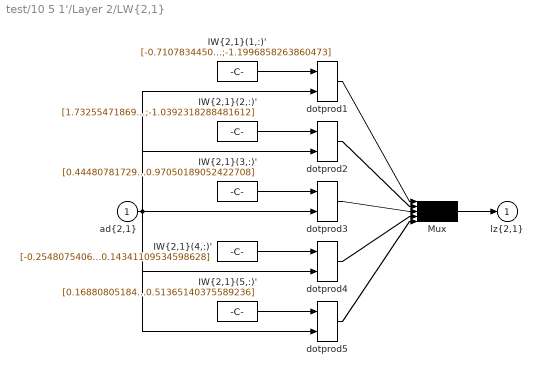
== system test/10 5 1'/Layer 2/LW{2,1} ==
  "ad{2,1}" : Inport  PortDimensions=10
  "IW{2,1}(1,:)'" : Constant  Value=[-0.71078344507396352;0.30081002804642054;-1.1363641709713621;-0.97347533252696283;-0.5979277345875148;-0.99192627483420337;0.91795932243561973;0.22559501980173671;1.1172099252626633;-1.1996858263860473]
      mask Display: disp('weights')
  "IW{2,1}(2,:)'" : Constant  Value=[1.7325547186980883;2.2857180727291828;-0.78754587876802318;1.5444556786858352;0.84052233791474307;2.6066696629566382;-0.60034170928796438;-1.3402571720122987;0.95127162068085203;-1.0392318288481612]
      mask Display: disp('weights')
  "IW{2,1}(3,:)'" : Constant  Value=[0.44480781729286578;0.5157077379354128;0.55457734738630893;0.91069851407073643;-0.32259065610010346;0.44670103955297219;0.87895630410635583;-0.28108644891413076;-0.59147187098635201;-0.97050189052422708]
      mask Display: disp('weights')
  "IW{2,1}(4,:)'" : Constant  Value=[-0.2548075406228747;0.2956991428149906;1.026624057927394;1.2712659563621749;0.58558175207289542;0.30524231453118134;-0.31501125369667471;-0.51240793303632637;-1.2915059625039966;0.14341109534598628]
      mask Display: disp('weights')
  "IW{2,1}(5,:)'" : Constant  Value=[0.16880805184704453;0.20115931124066974;-1.2643596506196184;-0.38871441001250534;-0.39612711338568368;-1.5506719715400121;-0.72119263107970766;-0.36878618292746607;-0.52983003236037307;0.51365140375589236]
      mask Display: disp('weights')
  Mux : Mux  Inputs=5
  dotprod{1..5} (5 alike) : neural/Weight Functions/dotprod  SystemSampleTime=-1
  "lz{2,1}" : Outport
  wires:
  Mux/1 -> "lz{2,1}"/1
  dotprod5/1 -> Mux/5
  "IW{2,1}(5,:)'"/1 -> dotprod5/1
  dotprod4/1 -> Mux/4
  "IW{2,1}(4,:)'"/1 -> dotprod4/1
  dotprod3/1 -> Mux/3
  "IW{2,1}(3,:)'"/1 -> dotprod3/1
  dotprod2/1 -> Mux/2
  "IW{2,1}(2,:)'"/1 -> dotprod2/1
  dotprod1/1 -> Mux/1
  "ad{2,1}"/1 -> dotprod5/2, dotprod4/2, dotprod3/2, dotprod2/2, dotprod1/2
  "IW{2,1}(1,:)'"/1 -> dotprod1/1

== system test/10 5 1'/Layer 3/Delays 1 ==
  "p{3}" : Inport  PortDimensions=5
  mux : Mux  Inputs=1
  "pd{3,2}" : Outport
  wires:
  mux/1 -> "pd{3,2}"/1
  "p{3}"/1 -> mux/1

== system test/10 5 1'/Layer 3/LW{3,2} ==
  "ad{3,2}" : Inport  PortDimensions=5
  "IW{3,2}(1,:)'" : Constant  Value=[0.2639106270038899;0.054598501385363873;-0.40979947985074278;-0.060659009105328857;0.29921056128475876]
      mask Display: disp('weights')
  Mux : Mux  Inputs=1
  dotprod1 : neural/Weight Functions/dotprod  SystemSampleTime=-1
  "lz{3,2}" : Outport
  wires:
  Mux/1 -> "lz{3,2}"/1
  dotprod1/1 -> Mux/1
  "ad{3,2}"/1 -> dotprod1/2
  "IW{3,2}(1,:)'"/1 -> dotprod1/1

== system test/Neural Network/Layer 1/Delays 1 ==
  "p{1}" : Inport  PortDimensions=3
  mux : Mux  Inputs=1
  "pd{1,1}" : Outport
  wires:
  "p{1}"/1 -> mux/1
  mux/1 -> "pd{1,1}"/1

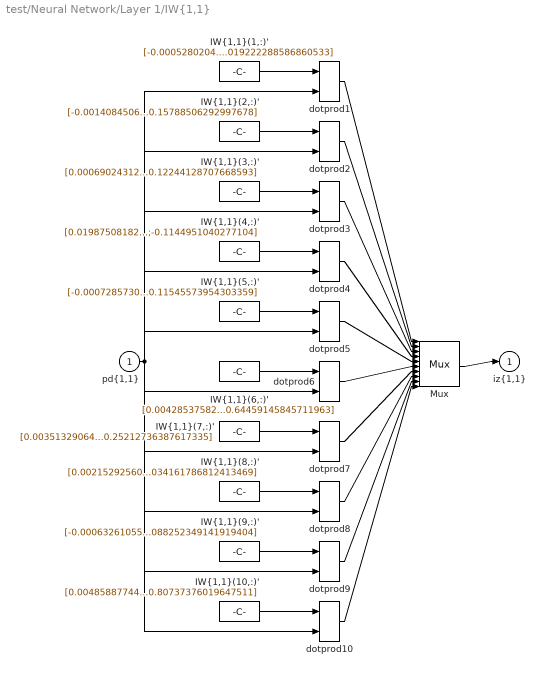
== system test/Neural Network/Layer 1/IW{1,1} ==
  "pd{1,1}" : Inport  PortDimensions=3
  "IW{1,1}(1,:)'" : Constant  Value=[-0.00052802041700726675;0.1894061234069748;0.019222288586860533]
      mask Display: disp('weights')
  "IW{1,1}(10,:)'" : Constant  Value=[0.0048588774473831767;-0.16914125105788577;-0.80737376019647511]
      mask Display: disp('weights')
  "IW{1,1}(2,:)'" : Constant  Value=[-0.0014084506052866039;0.92129809585440436;0.15788506292997678]
      mask Display: disp('weights')
  "IW{1,1}(3,:)'" : Constant  Value=[0.00069024312199982159;-0.17321471833168936;-0.12244128707668593]
      mask Display: disp('weights')
  "IW{1,1}(4,:)'" : Constant  Value=[0.019875081829974984;0.20457889337192051;-0.1144951040277104]
      mask Display: disp('weights')
  "IW{1,1}(5,:)'" : Constant  Value=[-0.0007285730411572788;0.8046058930501655;0.11545573954303359]
      mask Display: disp('weights')
  "IW{1,1}(6,:)'" : Constant  Value=[0.004285375826429948;-0.36528484988977361;-0.64459145845711963]
      mask Display: disp('weights')
  "IW{1,1}(7,:)'" : Constant  Value=[0.0035132906450386823;-0.24309288178463309;-0.25212736387617335]
      mask Display: disp('weights')
  "IW{1,1}(8,:)'" : Constant  Value=[0.0021529256068482019;0.34299757302654033;0.0034161786812413469]
      mask Display: disp('weights')
  "IW{1,1}(9,:)'" : Constant  Value=[-0.00063261055828300308;0.72925250001182806;0.0088252349141919404]
      mask Display: disp('weights')
  Mux : Mux  Inputs=10
  dotprod{1..10} (10 alike) : neural/Weight Functions/dotprod  SystemSampleTime=-1
  "iz{1,1}" : Outport
  wires:
  "IW{1,1}(1,:)'"/1 -> dotprod1/1
  "pd{1,1}"/1 -> dotprod1/2, dotprod2/2, dotprod3/2, dotprod4/2, dotprod5/2, dotprod6/2, dotprod7/2, dotprod8/2, dotprod9/2, dotprod10/2
  dotprod1/1 -> Mux/1
  "IW{1,1}(2,:)'"/1 -> dotprod2/1
  dotprod2/1 -> Mux/2
  "IW{1,1}(3,:)'"/1 -> dotprod3/1
  dotprod3/1 -> Mux/3
  "IW{1,1}(4,:)'"/1 -> dotprod4/1
  dotprod4/1 -> Mux/4
  "IW{1,1}(5,:)'"/1 -> dotprod5/1
  dotprod5/1 -> Mux/5
  "IW{1,1}(6,:)'"/1 -> dotprod6/1
  dotprod6/1 -> Mux/6
  "IW{1,1}(7,:)'"/1 -> dotprod7/1
  dotprod7/1 -> Mux/7
  "IW{1,1}(8,:)'"/1 -> dotprod8/1
  dotprod8/1 -> Mux/8
  "IW{1,1}(9,:)'"/1 -> dotprod9/1
  dotprod9/1 -> Mux/9
  "IW{1,1}(10,:)'"/1 -> dotprod10/1
  dotprod10/1 -> Mux/10
  Mux/1 -> "iz{1,1}"/1

== system test/Neural Network/Layer 2/Delays 1 ==
  "p{2}" : Inport  PortDimensions=10
  mux : Mux  Inputs=1
  "pd{2,1}" : Outport
  wires:
  "p{2}"/1 -> mux/1
  mux/1 -> "pd{2,1}"/1

== system test/Neural Network/Layer 2/LW{2,1} ==
  "ad{2,1}" : Inport  PortDimensions=10
  "IW{2,1}(1,:)'" : Constant  Value=[-0.55015410069137793;-0.010618623259439432;0.027966594983661702;-0.0014524855634991814;-0.19064518688694806;-0.053777706426675106;-0.00092308967994013695;0.41105097613450836;0.27453447204958775;0.34455833637583516]
      mask Display: disp('weights')
  Mux : Mux  Inputs=1
  dotprod1 : neural/Weight Functions/dotprod  SystemSampleTime=-1
  "lz{2,1}" : Outport
  wires:
  "IW{2,1}(1,:)'"/1 -> dotprod1/1
  "ad{2,1}"/1 -> dotprod1/2
  dotprod1/1 -> Mux/1
  Mux/1 -> "lz{2,1}"/1

== system test/Neural Network1/Layer 1/Delays 1 ==
  "p{1}" : Inport  PortDimensions=3
  mux : Mux  Inputs=1
  "pd{1,1}" : Outport
  wires:
  "p{1}"/1 -> mux/1
  mux/1 -> "pd{1,1}"/1

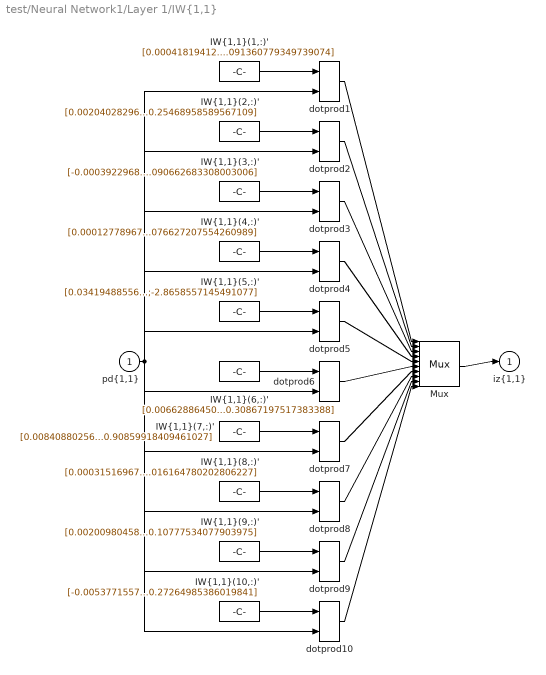
== system test/Neural Network1/Layer 1/IW{1,1} ==
  "pd{1,1}" : Inport  PortDimensions=3
  "IW{1,1}(1,:)'" : Constant  Value=[0.00041819412487026489;0.19176805747423262;-0.091360779349739074]
      mask Display: disp('weights')
  "IW{1,1}(10,:)'" : Constant  Value=[-0.005377155735325663;1.6719264422652267;-0.27264985386019841]
      mask Display: disp('weights')
  "IW{1,1}(2,:)'" : Constant  Value=[0.0020402829676183691;0.79391453282208213;-0.25468958589567109]
      mask Display: disp('weights')
  "IW{1,1}(3,:)'" : Constant  Value=[-0.00039229680356832059;-0.18619883738142878;0.090662683308003006]
      mask Display: disp('weights')
  "IW{1,1}(4,:)'" : Constant  Value=[0.00012778967431131456;-0.59877488070330998;-0.0076627207554260989]
      mask Display: disp('weights')
  "IW{1,1}(5,:)'" : Constant  Value=[0.034194885560356825;-0.97054893776829221;-2.8658557145491077]
      mask Display: disp('weights')
  "IW{1,1}(6,:)'" : Constant  Value=[0.0066288645047598016;-0.59220451719586786;-0.30867197517383388]
      mask Display: disp('weights')
  "IW{1,1}(7,:)'" : Constant  Value=[0.0084088025683557114;-1.3005230183008416;-0.90859918409461027]
      mask Display: disp('weights')
  "IW{1,1}(8,:)'" : Constant  Value=[0.00031516967825569517;0.049562210562956482;-0.016164780202806227]
      mask Display: disp('weights')
  "IW{1,1}(9,:)'" : Constant  Value=[0.0020098045886485921;-1.6895915011581817;-0.10777534077903975]
      mask Display: disp('weights')
  Mux : Mux  Inputs=10
  dotprod{1..10} (10 alike) : neural/Weight Functions/dotprod  SystemSampleTime=-1
  "iz{1,1}" : Outport
  wires:
  "IW{1,1}(1,:)'"/1 -> dotprod1/1
  "pd{1,1}"/1 -> dotprod1/2, dotprod2/2, dotprod3/2, dotprod4/2, dotprod5/2, dotprod6/2, dotprod7/2, dotprod8/2, dotprod9/2, dotprod10/2
  dotprod1/1 -> Mux/1
  "IW{1,1}(2,:)'"/1 -> dotprod2/1
  dotprod2/1 -> Mux/2
  "IW{1,1}(3,:)'"/1 -> dotprod3/1
  dotprod3/1 -> Mux/3
  "IW{1,1}(4,:)'"/1 -> dotprod4/1
  dotprod4/1 -> Mux/4
  "IW{1,1}(5,:)'"/1 -> dotprod5/1
  dotprod5/1 -> Mux/5
  "IW{1,1}(6,:)'"/1 -> dotprod6/1
  dotprod6/1 -> Mux/6
  "IW{1,1}(7,:)'"/1 -> dotprod7/1
  dotprod7/1 -> Mux/7
  "IW{1,1}(8,:)'"/1 -> dotprod8/1
  dotprod8/1 -> Mux/8
  "IW{1,1}(9,:)'"/1 -> dotprod9/1
  dotprod9/1 -> Mux/9
  "IW{1,1}(10,:)'"/1 -> dotprod10/1
  dotprod10/1 -> Mux/10
  Mux/1 -> "iz{1,1}"/1

== system test/Neural Network1/Layer 2/Delays 1 ==
  "p{2}" : Inport  PortDimensions=10
  mux : Mux  Inputs=1
  "pd{2,1}" : Outport
  wires:
  "p{2}"/1 -> mux/1
  mux/1 -> "pd{2,1}"/1

== system test/Neural Network1/Layer 2/LW{2,1} ==
  "ad{2,1}" : Inport  PortDimensions=10
  "IW{2,1}(1,:)'" : Constant  Value=[8.7426856941869087;0.045192338712173118;8.5291090890475711;-0.29260878738511342;-0.0045327532101514514;0.036215677132396117;0.030015335278148748;0.47010680194433208;0.027012593803511741;-0.76979211427053695]
      mask Display: disp('weights')
  Mux : Mux  Inputs=1
  dotprod1 : neural/Weight Functions/dotprod  SystemSampleTime=-1
  "lz{2,1}" : Outport
  wires:
  "IW{2,1}(1,:)'"/1 -> dotprod1/1
  "ad{2,1}"/1 -> dotprod1/2
  dotprod1/1 -> Mux/1
  Mux/1 -> "lz{2,1}"/1

== system test/Neural Network2/Layer 1/Delays 1 ==
  "p{1}" : Inport  PortDimensions=3
  mux : Mux  Inputs=1
  "pd{1,1}" : Outport
  wires:
  mux/1 -> "pd{1,1}"/1
  "p{1}"/1 -> mux/1

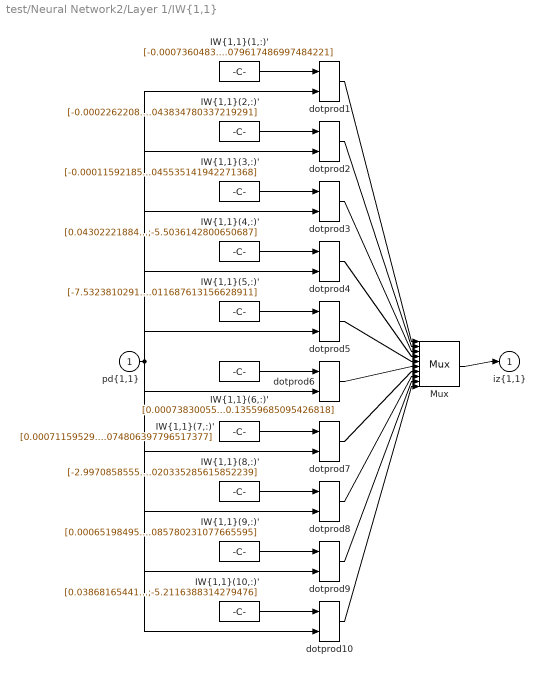
== system test/Neural Network2/Layer 1/IW{1,1} ==
  "pd{1,1}" : Inport  PortDimensions=3
  "IW{1,1}(1,:)'" : Constant  Value=[-0.00073604831665818394;-0.21927349118353281;0.079617486997484221]
      mask Display: disp('weights')
  "IW{1,1}(10,:)'" : Constant  Value=[0.038681654419164949;-2.0891745995145827;-5.2116388314279476]
      mask Display: disp('weights')
  "IW{1,1}(2,:)'" : Constant  Value=[-0.00022622083530015482;-0.21958545672772226;0.043834780337219291]
      mask Display: disp('weights')
  "IW{1,1}(3,:)'" : Constant  Value=[-0.00011592185121994382;-0.027016779101824633;-0.0045535141942271368]
      mask Display: disp('weights')
  "IW{1,1}(4,:)'" : Constant  Value=[0.043022218843091042;-2.5529296222639677;-5.5036142800650687]
      mask Display: disp('weights')
  "IW{1,1}(5,:)'" : Constant  Value=[-7.5323810291743923e-005;-0.013333927146165558;-0.011687613156628911]
      mask Display: disp('weights')
  "IW{1,1}(6,:)'" : Constant  Value=[0.00073830055057828208;0.27184799599198911;-0.13559685095426818]
      mask Display: disp('weights')
  "IW{1,1}(7,:)'" : Constant  Value=[0.00071159529576655532;0.20903678272143322;-0.074806397796517377]
      mask Display: disp('weights')
  "IW{1,1}(8,:)'" : Constant  Value=[-2.9970858555403793e-005;-0.00083104367468072563;-0.020335285615852239]
      mask Display: disp('weights')
  "IW{1,1}(9,:)'" : Constant  Value=[0.00065198495673468354;0.14845868031368067;-0.085780231077665595]
      mask Display: disp('weights')
  Mux : Mux  Inputs=10
  dotprod{1..10} (10 alike) : neural/Weight Functions/dotprod  SystemSampleTime=-1
  "iz{1,1}" : Outport
  wires:
  Mux/1 -> "iz{1,1}"/1
  dotprod10/1 -> Mux/10
  "IW{1,1}(10,:)'"/1 -> dotprod10/1
  dotprod9/1 -> Mux/9
  "IW{1,1}(9,:)'"/1 -> dotprod9/1
  dotprod8/1 -> Mux/8
  "IW{1,1}(8,:)'"/1 -> dotprod8/1
  dotprod7/1 -> Mux/7
  "IW{1,1}(7,:)'"/1 -> dotprod7/1
  dotprod6/1 -> Mux/6
  "IW{1,1}(6,:)'"/1 -> dotprod6/1
  dotprod5/1 -> Mux/5
  "IW{1,1}(5,:)'"/1 -> dotprod5/1
  dotprod4/1 -> Mux/4
  "IW{1,1}(4,:)'"/1 -> dotprod4/1
  dotprod3/1 -> Mux/3
  "IW{1,1}(3,:)'"/1 -> dotprod3/1
  dotprod2/1 -> Mux/2
  "IW{1,1}(2,:)'"/1 -> dotprod2/1
  dotprod1/1 -> Mux/1
  "pd{1,1}"/1 -> dotprod10/2, dotprod9/2, dotprod8/2, dotprod7/2, dotprod6/2, dotprod5/2, dotprod4/2, dotprod3/2, dotprod2/2, dotprod1/2
  "IW{1,1}(1,:)'"/1 -> dotprod1/1

== system test/Neural Network2/Layer 2/Delays 1 ==
  "p{2}" : Inport  PortDimensions=10
  mux : Mux  Inputs=1
  "pd{2,1}" : Outport
  wires:
  mux/1 -> "pd{2,1}"/1
  "p{2}"/1 -> mux/1

== system test/Neural Network2/Layer 2/LW{2,1} ==
  "ad{2,1}" : Inport  PortDimensions=10
  "IW{2,1}(1,:)'" : Constant  Value=[3.2472824622341632;-0.30984924542912556;-5.0441787284128852;-0.036084875466447577;7.5637899615500164;0.13585866916485631;3.5020245338726652;-3.1881810686250951;0.39393731951744249;-0.017325988582324838]
      mask Display: disp('weights')
  Mux : Mux  Inputs=1
  dotprod1 : neural/Weight Functions/dotprod  SystemSampleTime=-1
  "lz{2,1}" : Outport
  wires:
  Mux/1 -> "lz{2,1}"/1
  dotprod1/1 -> Mux/1
  "ad{2,1}"/1 -> dotprod1/2
  "IW{2,1}(1,:)'"/1 -> dotprod1/1

== system test/Neural Network3/Layer 1/Delays 1 ==
  "p{1}" : Inport  PortDimensions=3
  mux : Mux  Inputs=1
  "pd{1,1}" : Outport
  wires:
  mux/1 -> "pd{1,1}"/1
  "p{1}"/1 -> mux/1

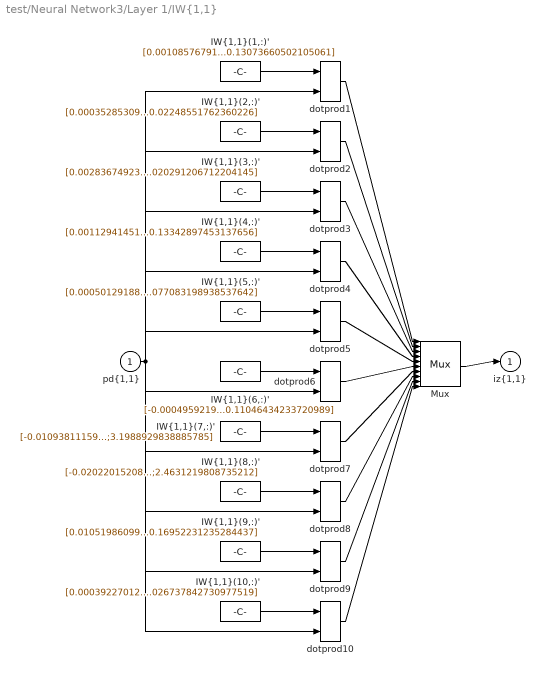
== system test/Neural Network3/Layer 1/IW{1,1} ==
  "pd{1,1}" : Inport  PortDimensions=3
  "IW{1,1}(1,:)'" : Constant  Value=[0.0010857679138187065;0.36340960837776604;-0.13073660502105061]
      mask Display: disp('weights')
  "IW{1,1}(10,:)'" : Constant  Value=[0.00039227012075212283;0.14436640771165141;-0.026737842730977519]
      mask Display: disp('weights')
  "IW{1,1}(2,:)'" : Constant  Value=[0.00035285309774959545;0.1285874218840449;-0.02248551762360226]
      mask Display: disp('weights')
  "IW{1,1}(3,:)'" : Constant  Value=[0.0028367492374543365;0.014705994298554431;0.020291206712204145]
      mask Display: disp('weights')
  "IW{1,1}(4,:)'" : Constant  Value=[0.0011294145174171248;0.37267136283476732;-0.13342897453137656]
      mask Display: disp('weights')
  "IW{1,1}(5,:)'" : Constant  Value=[0.00050129188642980028;0.026030725005333127;-0.077083198938537642]
      mask Display: disp('weights')
  "IW{1,1}(6,:)'" : Constant  Value=[-0.00049592198090705336;-0.20845595939141986;0.11046434233720989]
      mask Display: disp('weights')
  "IW{1,1}(7,:)'" : Constant  Value=[-0.010938111599835917;2.8312426045225956;3.1988929838885785]
      mask Display: disp('weights')
  "IW{1,1}(8,:)'" : Constant  Value=[-0.020220152089449241;2.7453027351882717;2.4631219808735212]
      mask Display: disp('weights')
  "IW{1,1}(9,:)'" : Constant  Value=[0.010519860996629986;0.31194762458033914;-0.16952231235284437]
      mask Display: disp('weights')
  Mux : Mux  Inputs=10
  dotprod{1..10} (10 alike) : neural/Weight Functions/dotprod  SystemSampleTime=-1
  "iz{1,1}" : Outport
  wires:
  Mux/1 -> "iz{1,1}"/1
  dotprod10/1 -> Mux/10
  "IW{1,1}(10,:)'"/1 -> dotprod10/1
  dotprod9/1 -> Mux/9
  "IW{1,1}(9,:)'"/1 -> dotprod9/1
  dotprod8/1 -> Mux/8
  "IW{1,1}(8,:)'"/1 -> dotprod8/1
  dotprod7/1 -> Mux/7
  "IW{1,1}(7,:)'"/1 -> dotprod7/1
  dotprod6/1 -> Mux/6
  "IW{1,1}(6,:)'"/1 -> dotprod6/1
  dotprod5/1 -> Mux/5
  "IW{1,1}(5,:)'"/1 -> dotprod5/1
  dotprod4/1 -> Mux/4
  "IW{1,1}(4,:)'"/1 -> dotprod4/1
  dotprod3/1 -> Mux/3
  "IW{1,1}(3,:)'"/1 -> dotprod3/1
  dotprod2/1 -> Mux/2
  "IW{1,1}(2,:)'"/1 -> dotprod2/1
  dotprod1/1 -> Mux/1
  "pd{1,1}"/1 -> dotprod10/2, dotprod9/2, dotprod8/2, dotprod7/2, dotprod6/2, dotprod5/2, dotprod4/2, dotprod3/2, dotprod2/2, dotprod1/2
  "IW{1,1}(1,:)'"/1 -> dotprod1/1

== system test/Neural Network3/Layer 2/Delays 1 ==
  "p{2}" : Inport  PortDimensions=10
  mux : Mux  Inputs=1
  "pd{2,1}" : Outport
  wires:
  mux/1 -> "pd{2,1}"/1
  "p{2}"/1 -> mux/1

== system test/Neural Network3/Layer 2/LW{2,1} ==
  "ad{2,1}" : Inport  PortDimensions=10
  "IW{2,1}(1,:)'" : Constant  Value=[3.3891104240580758;3.7377018358726533;0.10185800226630323;-3.1670320603710413;0.21800320871281928;0.40032879929123871;0.349246063274051;-0.002214043655877386;0.041853102349053241;-3.0078261477456332]
      mask Display: disp('weights')
  Mux : Mux  Inputs=1
  dotprod1 : neural/Weight Functions/dotprod  SystemSampleTime=-1
  "lz{2,1}" : Outport
  wires:
  Mux/1 -> "lz{2,1}"/1
  dotprod1/1 -> Mux/1
  "ad{2,1}"/1 -> dotprod1/2
  "IW{2,1}(1,:)'"/1 -> dotprod1/1
